simulink model "OneRobot_CT_S_PD"  (R2014b)
settings: Solver=ode45  StartTime=0.3  StopTime=10  FixedStep=0.01  RelTol=1e-3
settings Model: Creator=mshahria  LastModifiedBy=mshahria

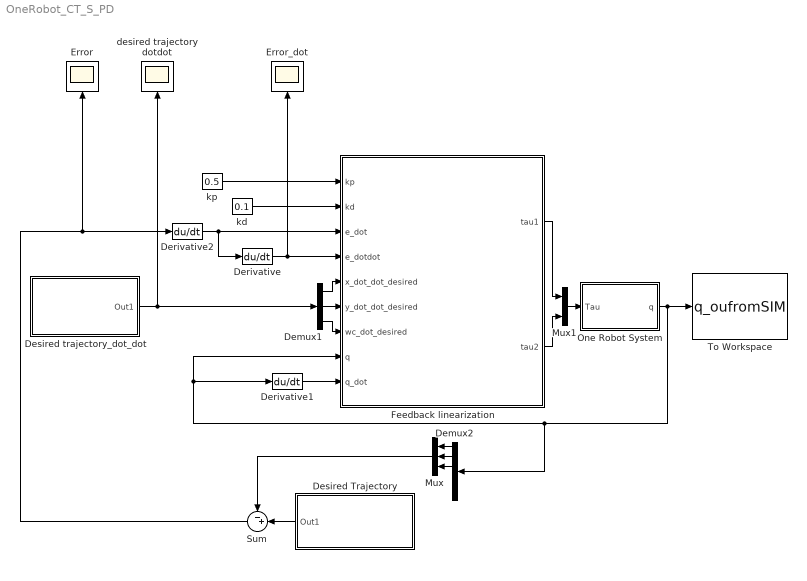
== system OneRobot_CT_S_PD ==
  " Error_dot" : Scope
  " One Robot System" : Subsystem
  Demux1 : Demux  Outputs=3
  Demux2 : Demux  Outputs=6
  Derivative : Derivative
  Derivative1 : Derivative
  Derivative2 : Derivative
  Desired Trajectory : Subsystem
  Desired trajectory_dot_dot : Subsystem
  Error : Scope
      settings: SaveName=ScopeData2
  "Feedback linearization " : MATLAB Function  TreatAsAtomicUnit=on
  Mux : Mux  Inputs=3
  Mux1 : Mux  Inputs=2
  Sum : Sum  Inputs=-+|
  To Workspace : ToWorkspace  VariableName=q_oufromSIM  SampleTime=-1
  desired trajectory dotdot : Scope
  kd : Constant  Value=0.1
  kp : Constant  Value=0.5
  wires:
  " One Robot System"/1(q) -> Demux2/1, "Feedback linearization "/8(q), Derivative1/1, To Workspace/1
  Derivative1/1 -> "Feedback linearization "/9(q_dot)
  "Feedback linearization "/1(tau1) -> Mux1/1
  "Feedback linearization "/2(tau2) -> Mux1/2
  Mux1/1 -> " One Robot System"/1(Tau)
  Demux1/3 -> "Feedback linearization "/7(wc_dot_desired)
  Demux1/2 -> "Feedback linearization "/6(y_dot_dot_desired)
  Demux1/1 -> "Feedback linearization "/5(x_dot_dot_desired)
  Demux2/1 -> Mux/1
  Demux2/2 -> Mux/2
  Demux2/3 -> Mux/3
  Mux/1 -> Sum/1
  kp/1 -> "Feedback linearization "/1(kp)
  kd/1 -> "Feedback linearization "/2(kd)
  Sum/1 -> Error/1, Derivative2/1
  Derivative/1 -> "Feedback linearization "/4(e_dotdot), " Error_dot"/1
  Desired trajectory_dot_dot/1(Out1) -> Demux1/1, desired trajectory dotdot/1
  Desired Trajectory/1(Out1) -> Sum/2
  Derivative2/1 -> Derivative/1, "Feedback linearization "/3(e_dot)

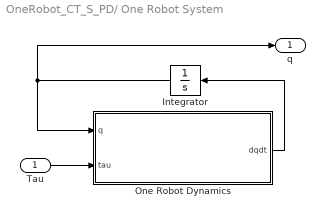
== system OneRobot_CT_S_PD/ One Robot System ==
  Tau : Inport
  Integrator : Integrator  InitialCondition=|  LimitOutput=on  UpperSaturationLimit=[inf,inf,inf,0.4,0.4,0.5]  LowerSaturationLimit=[-inf,-inf,-inf,-0.4,-0.4,-0.5]
      | [.2136; 0.7015
      | ;pi/3;0;0;0]
  One Robot Dynamics : MATLAB Function  TreatAsAtomicUnit=on
  q : Outport
  wires:
  Integrator/1 -> q/1, One Robot Dynamics/1(q)
  One Robot Dynamics/1(dqdt) -> Integrator/1
  Tau/1 -> One Robot Dynamics/2(tau)

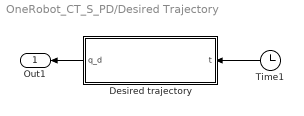
== system OneRobot_CT_S_PD/Desired Trajectory ==
  Desired trajectory : MATLAB Function  TreatAsAtomicUnit=on
  Time1 : Clock
  Out1 : Outport
  wires:
  Time1/1 -> Desired trajectory/1(t)
  Desired trajectory/1(q_d) -> Out1/1

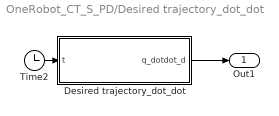
== system OneRobot_CT_S_PD/Desired trajectory_dot_dot ==
  Desired trajectory_dot_dot : MATLAB Function  TreatAsAtomicUnit=on
  Time2 : Clock
  Out1 : Outport
  wires:
  Time2/1 -> Desired trajectory_dot_dot/1(t)
  Desired trajectory_dot_dot/1(q_dotdot_d) -> Out1/1

== matlab function OneRobot_CT_S_PD/Desired Trajectory/Desired trajectory ==
  data: t input; q_d output
function q_d = fcn(t)

q_d = q_desired(t);

== matlab function OneRobot_CT_S_PD/ One Robot System/One Robot Dynamics ==
  data: dqdt output; q input; tau input
function dqdt= Robot_ode(q,tau)
dqdt=zeros(6,1);
% global tau_l tau_r; 
tau_l=tau(1);
tau_r=tau(2);

x_dot=q(4);
y_dot=q(5);
theta=q(3);
theta_dot=q(6);
q_dotdot = Qdotdot(tau_l,tau_r,theta,theta_dot,x_dot,y_dot);

dqdt(1)=q(4);
dqdt(2)=q(5);
dqdt(3)=q(6);
dqdt(4)=(q_dotdot(1));
dqdt(5)=(q_dotdot(2));
dqdt(6)=(q_dotdot(3));

== matlab function OneRobot_CT_S_PD/Feedback linearization  ==
  data: kp input; kd input; e_dot input; e_dotdot input; x_dot_dot_desired input; y_dot_dot_desired input; wc_dot_desired input; tau1 output; q input; q_dot input; tau2 output
function [tau1,tau2]= controller(kp,kd,e_dot,e_dotdot,x_dot_dot_desired,y_dot_dot_desired,wc_dot_desired,q,q_dot)

theta=q(3);
theta_dot=q(6);
x_dotdot=q_dot(4);
y_dotdot=q_dot(5);
theta_dotdot=q_dot(6);
x_dot=q(4);
y_dot=q(5);
vc=sqrt(x_dot^2+y_dot^2);
vc_dot_desired=sqrt(x_dot_dot_desired^2+y_dot_dot_desired^2);

u=kp*[sqrt(e_dot(1)^2+e_dot(2)^2);e_dot(3)]+ kd*[sqrt(e_dotdot(1)^2+e_dotdot(2)^2);e_dotdot(3)];


Tau= Tau_fdbckln(theta,theta_dot,vc,vc_dot_desired,wc_dot_desired)+ Hqfun(theta)*u;
tau1=Tau(1);
tau2=Tau(2);

== matlab function OneRobot_CT_S_PD/Desired trajectory_dot_dot/Desired trajectory_dot_dot ==
  data: t input; q_dotdot_d output
function q_dotdot_d = fcn(t)

q_dotdot_d = q_dotdot_desired(t);
